simulink model "Ej7"  (R2025a)
settings: Solver=VariableStepAuto  StartTime=0.0  StopTime=10.0  RelTol=1e-3
libraries: commrandsrc3 x1, dspfdesign x1
settings Model: Creator=Henry  LastModifiedBy=Henry

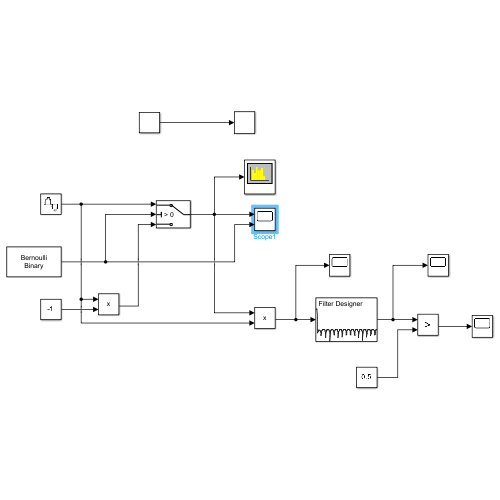
[thumbnail: Simulink's stored preview of the top-level diagram]
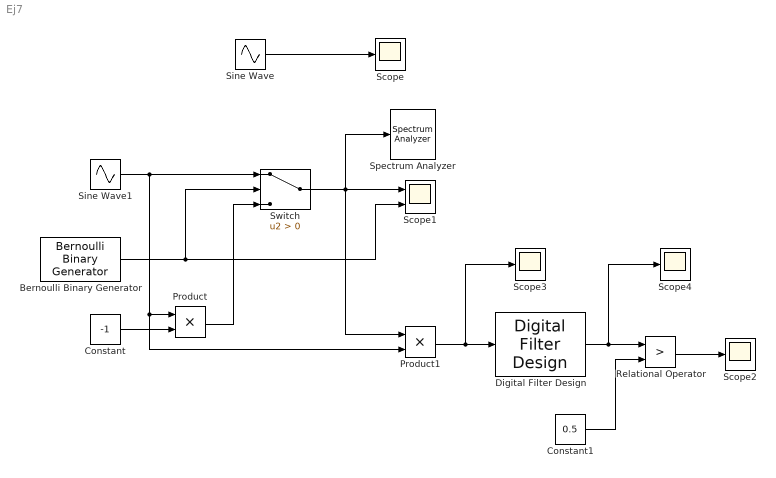
== system Ej7 ==
  Bernoulli Binary Generator : commrandsrc3/Bernoulli Binary Generator  ProbabilityOfZero=0.5  SeedSource=Auto  Seed=0  SampleTime=1  SamplesPerFrame=1  OutputDataType=double  SimulateUsing=Interpreted execution
  Constant : Constant  Value=-1
  Constant1 : Constant  Value=0.5
  Digital Filter Design : dspfdesign/Digital Filter Design  mwdsp_browser_bugfix_var=off
  Product : Product
  Product1 : Product
  Relational Operator : RelationalOperator  Operator=>  OutDataTypeStr=boolean  RndMeth=Simplest  InputSameDT=off
  Scope{,2..4} (4 alike) : Scope
      Scope settings: ActiveDisplayYMinimum=-1.2456318853205086  ActiveDisplayYMaximum=1.2490408795261734
      Scope2 settings: ActiveDisplayYMinimum=-1  ActiveDisplayYMaximum=1  DataLoggingVariableName=ScopeData2
      Scope3 settings: ActiveDisplayYMinimum=-1  ActiveDisplayYMaximum=1  DataLoggingVariableName=ScopeData3
      Scope4 settings: ActiveDisplayYMinimum=-0.8619660280553274  ActiveDisplayYMaximum=0.86196602805531941  DataLoggingVariableName=ScopeData4
  Scope1 : Scope  NumInputPorts=2
      settings: ActiveDisplayYMinimum=-1.2499999999999818  ActiveDisplayYMaximum=1.2499999999999918
  Sine Wave : Sin  SampleTime=0
  Sine Wave1 : Sin  Frequency=60*2*pi  SampleTime=0.0001
  Spectrum Analyzer : SpectrumAnalyzer  WindowPosition=[368.000000,182.000000,800.000000,500.000000,]  Visible=on  ScopeFrameLocation=window  WindowInvariantSamplesPerUpdate=on  YLimits=[-64.90282329902396 24.40994185909307]
  Switch : Switch  Criteria=u2 > Threshold  SaturateOnIntegerOverflow=off  InputSameDT=off
  wires:
  Sine Wave/1 -> Scope/1
  Sine Wave1/1 -> Product1/2, Product/1, Switch/1
  Bernoulli Binary Generator/1 -> Scope1/2, Switch/2
  Switch/1 -> Product1/1, Spectrum Analyzer/1, Scope1/1
  Constant/1 -> Product/2
  Product/1 -> Switch/3
  Product1/1 -> Scope3/1, Digital Filter Design/1
  Digital Filter Design/1 -> Scope4/1, Relational Operator/1
  Constant1/1 -> Relational Operator/2
  Relational Operator/1 -> Scope2/1
